simulink model "CNcs5"  (Simulink 6.2)
settings: Solver=ode4  SolverMode=SingleTasking  StartTime=0.0  StopTime=5  FixedStep=0.001  MaxStep=0.001  RelTol=1e-3  AbsTol=1e-3
undefined symbols (not defined in the file): alexlaw, bs_onoff, bs_scale, bsfsacrit, bsfsvcrit, cnsgain, fs_onoff, fs_scale, fsdelaycalc, ltdrk, phasicgain, pmcgain, pmctau2, pmctau3, saccrefract, saccsw, spgain, tonicgain, tvrD, tvrN, velnoise, velreconsw
libraries: simulink_extras x38, simulink x2
(part 1 of 5)
settings Model: Creator=jacobs  LastModifiedBy=jacobs  ExtModeAutoUpdateStatusClock=off
settings DataIOCC: LimitDataPoints=off  SaveOutput=off  SaveTime=off
settings OptimizationCC: BlockReduction=off  BooleanDataType=off
settings HardwareCC: TargetUnknown=on
settings STFCustomTargetCC: TargetFcnLib=ansi_tfl_tmw.mat  GenFloatMathFcnCalls=ANSI_C  ModelReferenceCompliant=off  SystemTargetFile=grt.tlc

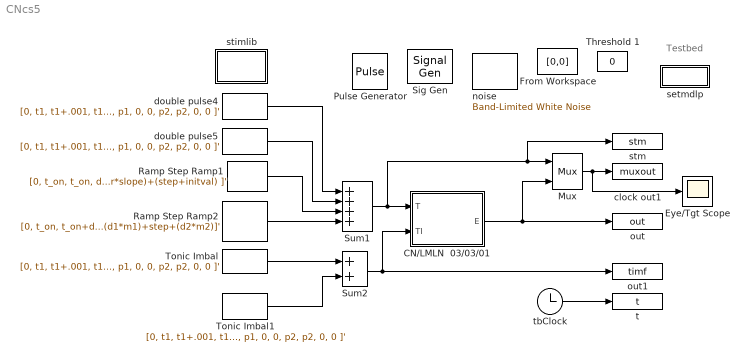
== system CNcs5 ==
  note: Testbed
  CN/LMLN  03/03/01 : Subsystem
      mask init:
      | k=0.25;loadmdlp;
      mask Display: disp('CN & LMLN\nModel')
  Eye/Tgt Scope : Scope
      settings: TickLabels=on  TimeRange=5  YMin=-5  YMax=32.5  DataFormat=Array
  From Workspace : FromWorkspace  VariableName=[0,0]
  Mux : Mux  Inputs=2
  Pulse Generator : DiscretePulseGenerator  PulseType=Time based  Amplitude=2  Period=.5  PulseWidth=100 * (.04)/(.5)  PhaseDelay=.1
  Ramp Step Ramp1 : FromWorkspace  VariableName=[0, t_on, t_on, dur+t_on dur+t_on; initval, initval, initval+step, (dur*slope)+(step+initval), (dur*slope)+(step+initval) ]'  mask{initval=0, t_on=1, step=0, dur=5, slope=0}
      mask prompts: initval "Initial value"; t_on "Time of step"; step "Size of step"; dur "Ramp duration"; slope "Ramp slope"
      mask help: Ramp Step Ramp
      mask Display: disp('Step\nRamp')
  Ramp Step Ramp2 : FromWorkspace  VariableName=[0, t_on, t_on+d1, t_on+d1, t_on+d1+d2, 10000; vi, vi, vi+(d1*m1), (vi+step)+(d1*m1), (vi+step)+(d1*m1)+(d2*m2), vi+(d1*m1)+step+(d2*m2)]'  mask{vi=0, t_on=.25, d1=4, m1=0, step=0, d2=2, m2=0}
      mask prompts: vi "Initial value"; t_on "Time of first ramp"; d1 "First Ramp duration"; m1 "First Ramp slope"; step "Size of step"; d2 "Second Ramp duration"; m2 "Second Ramp slope"
      mask help: Ramp Step Ramp
      mask Display: disp('Ramp\nStep\nRamp')
  Sig Gen : SignalGenerator  WaveForm=square  Amplitude=1.000000  Frequency=10.000000  Units=rad/sec
  Sum1 : Sum  Inputs=++++  SaturateOnIntegerOverflow=on  InputSameDT=on
  Sum2 : Sum  SaturateOnIntegerOverflow=on  InputSameDT=on
  Threshold 1 : Constant  Value=0
  Tonic Imbal : FromWorkspace  VariableName=[0, t1, t1+.001, t1+d1, t1+d1+.001, t1+d1+.001+ipd, t1+d1+.001+ipd, t1+d1+.001+ipd+d2, t1+d1+.001+ipd+d2, 10000; 0, 0, p1, p1, 0, 0, p2, p2, 0, 0 ]'  mask{@1=0, @2=0, @3=2, @4=0, @5=0, @6=3}
      mask prompts: @1 "Pulse 1 Magnitude"; @2 "Time of Pulse 1 Onset"; @3 "Pulse 1 Duration"; @4 "Interpulse Delay"; @5 "Pulse 2 Magnitude"; @6 "Pulse 2 Duration"
      mask help: Double Pulse
      mask init:
      | p1=@1; t1=@2; d1=@3; ipd=@4; p2=@5; d2=@6;
      mask Display: disp('Double\nPulse')
  Tonic Imbal1 : FromWorkspace  VariableName=[0, t1, t1+.001, t1+d1, t1+d1+.001, t1+d1+.001+ipd, t1+d1+.001+ipd, t1+d1+.001+ipd+d2, t1+d1+.001+ipd+d2, 10000; 0, 0, p1, p1, 0, 0, p2, p2, 0, 0 ]'  mask{@1=0, @2=0, @3=3.5, @4=0, @5=0, @6=1.5}
      mask prompts: @1 "Pulse 1 Magnitude"; @2 "Time of Pulse 1 Onset"; @3 "Pulse 1 Duration"; @4 "Interpulse Delay"; @5 "Pulse 2 Magnitude"; @6 "Pulse 2 Duration"
      mask help: Double Pulse
      mask init:
      | p1=@1; t1=@2; d1=@3; ipd=@4; p2=@5; d2=@6;
      mask Display: disp('Double\nPulse')
  clock out1 : ToWorkspace  VariableName=muxout  SaveFormat=Array
      settings: MaxDataPoints=100000
  double pulse4 : FromWorkspace  VariableName=[0, t1, t1+.001, t1+d1, t1+d1+.001, t1+d1+.001+ipd, t1+d1+.001+ipd, t1+d1+.001+ipd+d2, t1+d1+.001+ipd+d2, 10000; 0, 0, p1, p1, 0, 0, p2, p2, 0, 0 ]'  mask{@1=15, @2=2, @3=2, @4=0, @5=0, @6=5}
      mask prompts: @1 "Pulse 1 Magnitude"; @2 "Time of Pulse 1 Onset"; @3 "Pulse 1 Duration"; @4 "Interpulse Delay"; @5 "Pulse 2 Magnitude"; @6 "Pulse 2 Duration"
      mask help: Double Pulse
      mask init:
      | p1=@1; t1=@2; d1=@3; ipd=@4; p2=@5; d2=@6;
      mask Display: disp('Double\nPulse')
  double pulse5 : FromWorkspace  VariableName=[0, t1, t1+.001, t1+d1, t1+d1+.001, t1+d1+.001+ipd, t1+d1+.001+ipd, t1+d1+.001+ipd+d2, t1+d1+.001+ipd+d2, 10000; 0, 0, p1, p1, 0, 0, p2, p2, 0, 0 ]'  mask{@1=0, @2=0, @3=1, @4=0, @5=0, @6=4.5}
      mask prompts: @1 "Pulse 1 Magnitude"; @2 "Time of Pulse 1 Onset"; @3 "Pulse 1 Duration"; @4 "Interpulse Delay"; @5 "Pulse 2 Magnitude"; @6 "Pulse 2 Duration"
      mask help: Double Pulse
      mask init:
      | p1=@1; t1=@2; d1=@3; ipd=@4; p2=@5; d2=@6;
      mask Display: disp('Double\nPulse')
  noise : simulink/Sources/Band-Limited White Noise  Cov=[0.1]  Ts=0.1  seed=[23341]
  out : ToWorkspace  VariableName=out  SaveFormat=Array
      settings: MaxDataPoints=100000
  out1 : ToWorkspace  VariableName=timf  SaveFormat=Array
      settings: MaxDataPoints=100000
  setmdlp : Subsystem
      settings: OpenFcn=setmdlp
      mask Display: disp('setmdlp')
  stimlib : Subsystem
      settings: OpenFcn=stimlib
      mask Display: disp('Stimlib')
  stm : ToWorkspace  VariableName=stm  SaveFormat=Array
      settings: MaxDataPoints=100000
  t : ToWorkspace  VariableName=t  SaveFormat=Array
      mask init:
      | global t
      settings: MaxDataPoints=100000
  tbClock : Clock
      settings: Decimation=10
  wires:
  tbClock/1 -> t/1
  double pulse4/1 -> Sum1/1
  Sum1/1 -> CN/LMLN  03/03/01/1(T), stm/1, Mux/1
  CN/LMLN  03/03/01/1(E) -> out/1, Mux/2
  Mux/1 -> clock out1/1, Eye/Tgt Scope/1
  Tonic Imbal/1 -> Sum2/1
  Tonic Imbal1/1 -> Sum2/2
  Sum2/1 -> CN/LMLN  03/03/01/2(TI), out1/1
  double pulse5/1 -> Sum1/2
  Ramp Step Ramp1/1 -> Sum1/3
  Ramp Step Ramp2/1 -> Sum1/4

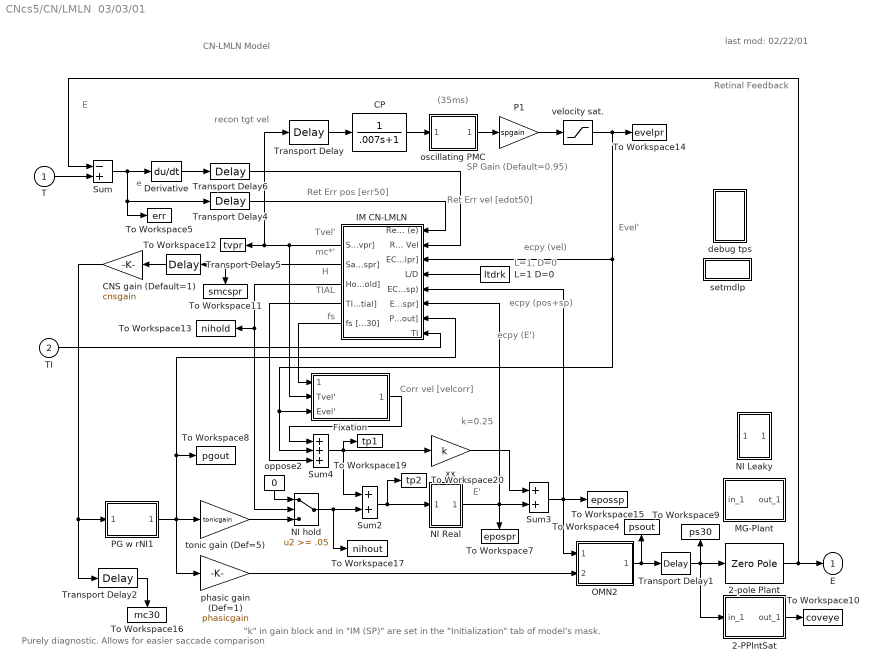
== system CNcs5/CN/LMLN  03/03/01 ==
  note: E'
  note: k=0.25
  note: "k" in gain block and in "IM (SP)" are set in
      | the "Initialization" tab of model's mask.
  note: E
  note: e
  note: TIAL
  note: H
  note: mc*'
  note: Tvel'
  note: ecpy
      | (E')
  note: ecpy (vel)
  note: (35ms)
  note: Retinal Feedback
  note: recon tgt vel
  note: last mod:
      | 02/22/01
  note: Evel'
  note: CN-LMLN Model
  note: ecpy
      | (pos+sp)
  note: Ret Err vel
      | [edot50]
  note: Ret Err pos [err50]
  note: Purely diagnostic.  Allows for easier
      | saccade comparison
  note: SP Gain
      | (Default=0.95)
  note: L=1, D=0
  note: Corr vel
      | [velcorr]
  note: fs
  T : Inport  Port=1  LatchInput=off
  TI : Inport  Port=2  LatchInput=off
  2-PPlntSat : Subsystem
      mask Display: disp('2-P Plant\n[Sat]')
  2-pole Plant : ZeroPole  Zeros=[ ]  Poles=[ -1/.18 -1/.007]  Gain=[1/.18 * 1/.007]
      mask Display: disp('2-pole\nPlant')
  CNS gain (Default=1) : Gain  Orientation=left  Gain=cnsgain  SaturateOnIntegerOverflow=on
  CP : TransferFcn  Denominator=[.007 1]
  Derivative : Derivative
      mask Display: disp('s')
  Fixation : Subsystem
      mask Display: disp('Fixation')
  IM CN-LMLN : Subsystem  Orientation=left
      mask Display: disp('IM\nCN-LMLN')
  L=1 D=0 : Constant  Orientation=left  Value=ltdrk
  MG-Plant : Subsystem
      mask Display: disp('MG Plant\n[K,tau,sat]')
  NI Leaky : Subsystem
      mask Display: disp('N\nLeaky')
  NI Real : Subsystem
      mask Display: disp('NI\nReal')
  NI hold : Switch  Threshold=.05  SaturateOnIntegerOverflow=on  InputSameDT=on
  OMN2 : Subsystem
      mask Display: disp('<--"tonic" \nOMN2\n<--"phasic"')
  P1 : Gain  Gain=spgain  SaturateOnIntegerOverflow=on
  PG w rNI1 : Subsystem
      mask Display: disp('PG rNI\n(2P)')
  Sum : Sum  Inputs=-+  SaturateOnIntegerOverflow=on  InputSameDT=on
  Sum2 : Sum  SaturateOnIntegerOverflow=on  InputSameDT=on
  Sum3 : Sum  SaturateOnIntegerOverflow=on  InputSameDT=on
  Sum4 : Sum  Inputs=+++  SaturateOnIntegerOverflow=on  InputSameDT=on
  To Workspace10 : ToWorkspace  VariableName=coveye  SaveFormat=Array
      settings: MaxDataPoints=10000
  To Workspace11 : ToWorkspace  VariableName=smcspr  SaveFormat=Array
      settings: Orientation=down  MaxDataPoints=10000
  To Workspace12 : ToWorkspace  VariableName=tvpr  SaveFormat=Array
      settings: MaxDataPoints=10000
  To Workspace13 : ToWorkspace  VariableName=nihold  SaveFormat=Array
      settings: MaxDataPoints=10000
  To Workspace14 : ToWorkspace  VariableName=evelpr  SaveFormat=Array
      settings: MaxDataPoints=10000
  To Workspace15 : ToWorkspace  VariableName=epossp  SaveFormat=Array
      settings: MaxDataPoints=10000
  To Workspace16 : ToWorkspace  VariableName=mc30  SaveFormat=Array
      settings: Orientation=down  MaxDataPoints=10000
  To Workspace17 : ToWorkspace  VariableName=nihout  SaveFormat=Array
      settings: MaxDataPoints=10000
  To Workspace19 : ToWorkspace  VariableName=tp1  SaveFormat=Array
      settings: MaxDataPoints=10000
  To Workspace20 : ToWorkspace  VariableName=tp2  SaveFormat=Array
      settings: MaxDataPoints=10000
  To Workspace4 : ToWorkspace  VariableName=psout  SaveFormat=Array
      settings: Orientation=up  MaxDataPoints=10000
  To Workspace5 : ToWorkspace  VariableName=err  SaveFormat=Array
      settings: MaxDataPoints=10000
  To Workspace7 : ToWorkspace  VariableName=epospr  SaveFormat=Array
      settings: Orientation=down  MaxDataPoints=10000
  To Workspace8 : ToWorkspace  VariableName=pgout  SaveFormat=Array
      settings: MaxDataPoints=10000
  To Workspace9 : ToWorkspace  VariableName=ps30  SaveFormat=Array
      settings: Orientation=up  MaxDataPoints=10000
  Transport Delay : TransportDelay  DelayTime=0.015
      mask Display: disp('15ms')
  Transport Delay1 : TransportDelay  DelayTime=0.03
      mask Display: disp('30ms')
  Transport Delay2 : TransportDelay  DelayTime=0.03
      mask Display: disp('30ms')
  Transport Delay4 : TransportDelay  DelayTime=.05
      mask Display: disp('50ms')
  Transport Delay5 : TransportDelay  Orientation=left  DelayTime=0.001
      mask Display: disp('1ms')
  Transport Delay6 : TransportDelay  DelayTime=.05
      mask Display: disp('50ms')
  debug tps : Subsystem
  oppose2 : Constant  Orientation=down  Value=0
  oscillating PMC : Subsystem
      mask Display: disp('PMC+')
  phasic gain (Def=1) : Gain  Gain=phasicgain  SaturateOnIntegerOverflow=on
  setmdlp : Subsystem
      settings: OpenFcn=setmdlp
      mask Display: disp('setmdlp')
  tonic gain (Def=5) : Gain  Gain=tonicgain  SaturateOnIntegerOverflow=on
  velocity sat. : Saturate  UpperLimit=90  LowerLimit=-90
  xx : Gain  Gain=k  SaturateOnIntegerOverflow=on
  E : Outport  InitialOutput=0
  wires:
  Derivative/1 -> Transport Delay6/1
  Sum/1 -> Derivative/1, Transport Delay4/1, To Workspace5/1
  T/1 -> Sum/2
  Transport Delay4/1 -> IM CN-LMLN/1(RetErr Pos (e))
  L=1 D=0/1 -> IM CN-LMLN/4(L/D)
  Transport Delay6/1 -> IM CN-LMLN/2(RetErr Vel)
  CP/1 -> oscillating PMC/1(desired eye vel)
  oscillating PMC/1(efference copy eye vel) -> P1/1
  Transport Delay/1 -> CP/1
  velocity sat./1 -> To Workspace14/1, IM CN-LMLN/3(ECPY [evelpr]), Fixation/3(Evel'), Sum4/2
  P1/1 -> velocity sat./1
  TI/1 -> IM CN-LMLN/8(TI)
  IM CN-LMLN/1(SPmc [tvpr]) -> To Workspace12/1, Transport Delay/1, Fixation/2(Tvel')
  Sum4/1 -> xx/1, Sum2/1, To Workspace19/1
  IM CN-LMLN/4(TIAL [tial]) -> Sum4/3
  PG w rNI1/1(PG [pgout]) -> IM CN-LMLN/7(PG [pgout]), To Workspace8/1, tonic gain (Def=5)/1, phasic gain (Def=1)/1
  2-pole Plant/1 -> E/1, Sum/1
  2-PPlntSat/1(out_1) -> To Workspace10/1
  Transport Delay1/1 -> 2-pole Plant/1, To Workspace9/1, 2-PPlntSat/1(in_1)
  OMN2/1("[psout]") -> To Workspace4/1, Transport Delay1/1
  Transport Delay2/1 -> To Workspace16/1
  tonic gain (Def=5)/1 -> NI hold/3
  phasic gain (Def=1)/1 -> OMN2/2("[pgout]")
  NI hold/1 -> Sum2/2, To Workspace17/1
  xx/1 -> Sum3/1
  NI Real/1(NIOUT [epospr]) -> Sum3/2, To Workspace7/1, IM CN-LMLN/6(ECPY [epospr])
  Sum3/1 -> IM CN-LMLN/5(ECPY (epossp)), To Workspace15/1, OMN2/1("[epossp]")
  Fixation/1(" CorrVel [velcorr]") -> Sum4/1
  Sum2/1 -> NI Real/1(PG + (TIAL+SP)), To Workspace20/1
  IM CN-LMLN/5(fs [fsmc30]) -> Fixation/1(fs [fsmc30])
  oppose2/1 -> NI hold/1
  IM CN-LMLN/3(Hold [nihold]) -> To Workspace13/1, NI hold/2
  IM CN-LMLN/2(Saccmc [smcspr]) -> To Workspace11/1, Transport Delay5/1
  CNS gain (Default=1)/1 -> PG w rNI1/1("[mcsprd]"), Transport Delay2/1
  Transport Delay5/1 -> CNS gain (Default=1)/1

== system CNcs5/setmdlp ==

== system CNcs5/stimlib ==

== system CNcs5/CN/LMLN  03/03/01/2-PPlntSat ==
  note: A 2-pole plant can be simulated by:
      | 1. no limitation on lateral gaze
      | 2. a hard limitation - placing a saturation in the plant [eg, 55 deg]
      | 3. a soft limitation - add the dead zone  [DZ slope>0]
  in_1 : Inport  Port=1  LatchInput=off
  2 pole : ZeroPole  Zeros=[ ]  Poles=[ -1/.18 -1/.007]  Gain=[1/.18 * 1/.007]
      mask Display: disp('2-pole\nPlant')
  DZ slope : Constant  Value=0.05
  Dead Zone : DeadZone  LowerValue=-55  UpperValue=55  SaturateOnIntegerOverflow=on
  Product : Product  SaturateOnIntegerOverflow=on  RndMeth=Zero  InputSameDT=on
  Saturation : Saturate  UpperLimit=55  LowerLimit=-55
  Sum3 : Sum  SaturateOnIntegerOverflow=on  InputSameDT=on
  out_1 : Outport  InitialOutput=0
  wires:
  DZ slope/1 -> Product/2
  Product/1 -> Sum3/2
  Sum3/1 -> out_1/1
  Saturation/1 -> Sum3/1
  Dead Zone/1 -> Product/1
  2 pole/1 -> Saturation/1, Dead Zone/1
  in_1/1 -> 2 pole/1

== system CNcs5/CN/LMLN  03/03/01/Fixation ==
  note: Fixation (counter-signal)
  note: Last mod: 02/22/01
  note: Positional error is passed through a gaussian-like function whose greatest
      | response occurs between +/-0.5 deg (approx), corresponding to the sensitivity
      | of the fovea.
  note: This factor is used (with an additional gain factor) to scale the velocity error,
      | which is then subtracted from the velocity signal that is sent from the
      | common neural integrator to the ocular motor neurons.
  note: This should have the effect of reducing the high velocity error (due
      | to CN oscillation or other sources) enough to permit an extension of
      | the foveation period.
  note: *Mod*
  fs [fsmc30] : Inport  Port=1  LatchInput=off
  Tvel' : Inport  Port=2  LatchInput=off
  Evel' : Inport  Port=3  LatchInput=off
  "30 " : Subsystem  mask{prolong=30}
      mask prompts: prolong "Prolong pulse by?  (msec)"
      mask Display: disp('prolong')
  Boolify2 : Subsystem
      mask Display: disp('Boolify')
  Product : Product  Inputs=3  SaturateOnIntegerOverflow=on  RndMeth=Zero  InputSameDT=on
  Product1 : Product  SaturateOnIntegerOverflow=on  RndMeth=Zero  InputSameDT=on
  Sum5 : Sum  Inputs=+-  SaturateOnIntegerOverflow=on  InputSameDT=on
  Transport Delay7 : TransportDelay  DelayTime=0.050
      mask Display: disp('50ms')
  Vel Sens Factor : Gain  Gain=4  SaturateOnIntegerOverflow=on
  WF % to be applied : Gain  SaturateOnIntegerOverflow=on
  on/off : Constant  Orientation=down
  position sensitivity W2 : Lookup  InputValues="[-5 -2  -1 -0.5   0.5   1    2    5]"  OutputValues="[ 0   0.125    0.5     1      1     0.5    0.125  0]"  SaturateOnIntegerOverflow=on
  t : ToWorkspace  VariableName=velfact  SaveFormat=Array
      mask init:
      | global t
      settings: MaxDataPoints=100000
  t2 : ToWorkspace  VariableName=velcorr  SaveFormat=Array
      mask init:
      | global t
      settings: MaxDataPoints=100000
  t3 : ToWorkspace  VariableName=fs30p  SaveFormat=Array
      mask init:
      | global t
      settings: MaxDataPoints=100000
  t4 : ToWorkspace  VariableName=nystagvel  SaveFormat=Array
      mask init:
      | global t
      settings: MaxDataPoints=100000
  velocity sensitivity N : Lookup  InputValues="[-20 -16  -12   -6  -4  4   6   12  16 20]"  OutputValues="[0 0   0.1    0.3    1   1   0.3  0.1   0 0]"  SaturateOnIntegerOverflow=on
  velocity sensitivity W2 : Lookup  InputValues="[-30 -15   -8  -4   4     8  15  30]"  OutputValues="[0  0.125   0.5    1    1    0.5   0.125  0]"  SaturateOnIntegerOverflow=on
  " CorrVel [velcorr]" : Outport  InitialOutput=0
  wires:
  Sum5/1 -> velocity sensitivity N/1, t4/1, WF % to be applied/1
  velocity sensitivity N/1 -> Vel Sens Factor/1, t/1
  Evel'/1 -> Sum5/2
  Tvel'/1 -> Transport Delay7/1
  Transport Delay7/1 -> Sum5/1
  WF % to be applied/1 -> Product/3
  Product/1 -> t2/1, Product1/2
  Product1/1 -> " CorrVel [velcorr]"/1
  on/off/1 -> Product1/1
  fs [fsmc30]/1 -> Boolify2/1(In1)
  Boolify2/1(Out1) -> "30 "/1(value(in))
  "30 "/1(value(out)) -> Product/1, t3/1
  Vel Sens Factor/1 -> Product/2

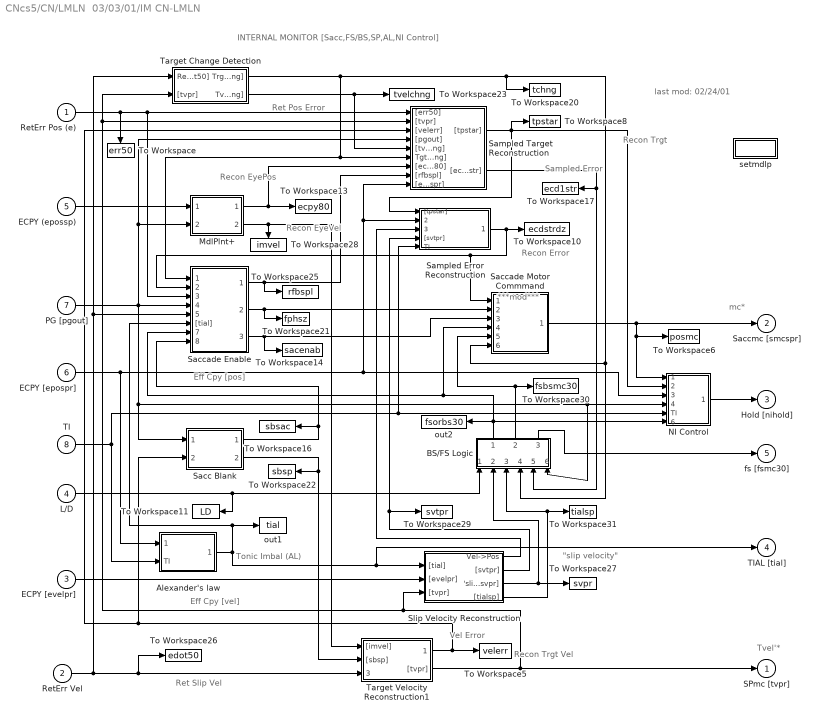
== system CNcs5/CN/LMLN  03/03/01/IM CN-LMLN ==
  note: INTERNAL MONITOR [Sacc,FS/BS,SP,AL,NI Control]
  note: last mod:
      | 02/24/01
  note: mc*
  note: Tvel'*
  note: "slip velocity"
  note: Recon
      | Trgt
  note: Recon
      | EyePos
  note: Recon
      | EyeVel
  note: Sampled
      | Error
  note: Recon Error
  note: Recon
      | Trgt Vel
  note: Vel
      | Error
  note: Eff Cpy [vel]
  note: Eff Cpy [pos]
  note: Tonic Imbal (AL)
  note: Ret Slip Vel
  note: Ret Pos Error
  note: ***mod***
  RetErr Pos (e) : Inport  Port=1  LatchInput=off
  RetErr Vel : Inport  Port=2  LatchInput=off
  ECPY [evelpr] : Inport  Port=3  LatchInput=off
  L/D : Inport  Port=4  LatchInput=off
  ECPY (epossp) : Inport  Port=5  LatchInput=off
  ECPY [epospr] : Inport  Port=6  LatchInput=off
  PG [pgout] : Inport  Port=7  LatchInput=off
  TI : Inport  Port=8  LatchInput=off
  Alexander's law : Subsystem  mask{slope=alexlaw}
      mask help: Alexander's Law
      mask Display: disp('Alexander''s\nLaw')
  BS/FS Logic : Subsystem  Orientation=up
      mask Display: disp('BS/FS\nLogic')
  MdlPlnt+ : Subsystem
      mask Display: disp('Model\nPlant+')
  NI Control : Subsystem
      mask Display: disp('NI\nControl')
  Sacc Blank : Subsystem
      mask Display: disp('Saccade\n& Drift\nBlanking')
  Saccade Enable : Subsystem
      mask Display: disp('Saccade\nEnable')
  Saccade Motor Commmand : Subsystem
      mask Display: disp('Saccade\nMotor\nCommand')
  Sampled Error Reconstruction : Subsystem
      mask Display: disp('Sampled Error\nReconstruction')
  Sampled Target Reconstruction : Subsystem
      mask Display: disp('Sampled\nTarget\nReconstruction')
  Slip Velocity Reconstruction : Subsystem
      mask Display: disp('Slip\nVelocity\nReconstruction')
  Target Change Detection : Subsystem
      mask Display: disp('Target Change\nDetection')
  Target Velocity Reconstruction1 : Subsystem
      mask Display: disp('Target\nVelocity\nReconstruction')
  To Workspace : ToWorkspace  VariableName=err50  SaveFormat=Array
      settings: Orientation=down  MaxDataPoints=10000
  To Workspace10 : ToWorkspace  VariableName=ecdstrdz  SaveFormat=Array
      settings: MaxDataPoints=10000
  To Workspace11 : ToWorkspace  VariableName=LD  SaveFormat=Array
      settings: MaxDataPoints=10000
  To Workspace13 : ToWorkspace  VariableName=ecpy80  SaveFormat=Array
      settings: MaxDataPoints=10000
  To Workspace14 : ToWorkspace  VariableName=sacenab  SaveFormat=Array
      settings: MaxDataPoints=10000
      mask Type: imsw1in
  To Workspace16 : ToWorkspace  VariableName=sbsac  SaveFormat=Array
      settings: MaxDataPoints=10000
  To Workspace17 : ToWorkspace  VariableName=ecd1str  SaveFormat=Array
      settings: MaxDataPoints=10000
  To Workspace20 : ToWorkspace  VariableName=tchng  SaveFormat=Array
      settings: MaxDataPoints=10000
  To Workspace21 : ToWorkspace  VariableName=fphsz  SaveFormat=Array
      settings: MaxDataPoints=10000
  To Workspace22 : ToWorkspace  VariableName=sbsp  SaveFormat=Array
      settings: MaxDataPoints=10000
  To Workspace23 : ToWorkspace  VariableName=tvelchng  SaveFormat=Array
      settings: MaxDataPoints=10000
  To Workspace25 : ToWorkspace  VariableName=rfbspl  SaveFormat=Array
      settings: MaxDataPoints=10000
      mask Type: imsw1in
  To Workspace26 : ToWorkspace  VariableName=edot50  SaveFormat=Array
      settings: MaxDataPoints=10000
  To Workspace27 : ToWorkspace  VariableName=svpr  SaveFormat=Array
      settings: MaxDataPoints=10000
  To Workspace28 : ToWorkspace  VariableName=imvel  SaveFormat=Array
      settings: Orientation=down  MaxDataPoints=10000
      mask Type: imsw1in
  To Workspace29 : ToWorkspace  VariableName=svtpr  SaveFormat=Array
      settings: MaxDataPoints=10000
  To Workspace30 : ToWorkspace  VariableName=fsbsmc30  SaveFormat=Array
      settings: MaxDataPoints=10000
  To Workspace31 : ToWorkspace  VariableName=tialsp  SaveFormat=Array
      settings: MaxDataPoints=10000
  To Workspace5 : ToWorkspace  VariableName=velerr  SaveFormat=Array
      settings: MaxDataPoints=10000
  To Workspace6 : ToWorkspace  VariableName=posmc  SaveFormat=Array
      settings: MaxDataPoints=10000
  To Workspace8 : ToWorkspace  VariableName=tpstar  SaveFormat=Array
      settings: MaxDataPoints=10000
  out1 : ToWorkspace  VariableName=tial  SaveFormat=Array
      settings: MaxDataPoints=100000
  out2 : ToWorkspace  VariableName=fsorbs30  SaveFormat=Array
      settings: MaxDataPoints=100000
  setmdlp : Subsystem
      settings: OpenFcn=setmdlp
      mask Display: disp('setmdlp')
  SPmc [tvpr] : Outport  InitialOutput=0
  Saccmc [smcspr] : Outport  Port=2  InitialOutput=0
  Hold [nihold] : Outport  Port=3  InitialOutput=0
  TIAL [tial] : Outport  Port=4  InitialOutput=0
  fs [fsmc30] : Outport  Port=5  InitialOutput=0
  wires:
  NI Control/1(Hold [nihold]) -> Hold [nihold]/1
  L/D/1 -> BS/FS Logic/1(L/D), To Workspace11/1
  ECPY [epospr]/1 -> Alexander's law/1(ECPY [epospr]), NI Control/3("[epospr]"), Sampled Error Reconstruction/2("[epospr]"), Sampled Target Reconstruction/9("[epospr]")
  TI/1 -> Alexander's law/2(TI), NI Control/5(TI), Sampled Error Reconstruction/5(TI)
  PG [pgout]/1 -> Sacc Blank/1(PG [pgout]), NI Control/4(PG [pgout]), BS/FS Logic/6("[pgout]"), Saccade Enable/4("[pgout]"), MdlPlnt+/2("[pgout]"), Sampled Target Reconstruction/4("[pgout]")
  ECPY (epossp)/1 -> MdlPlnt+/1("[epossp]")
  MdlPlnt+/2("[imvel]") -> To Workspace28/1, Target Velocity Reconstruction1/1("[imvel]")
  BS/FS Logic/1("[fsorbs30]") -> out2/1, Saccade Enable/7("[fsorbs30]"), Saccade Motor Commmand/4("[fsorbs30]"), NI Control/6("[fsorbs30]")
  Saccade Enable/2(FPh Size [fphsz]) -> To Workspace21/1, Saccade Motor Commmand/2("[fphsz]")
  Saccade Enable/3("[sacenab]") -> To Workspace14/1, Saccade Motor Commmand/3("[sacenab]")
  Saccade Enable/1("[rfbspl]") -> To Workspace25/1, Sampled Target Reconstruction/8("[rfbspl]")
  MdlPlnt+/1("[ecpy80]") -> Sampled Target Reconstruction/7("[ecpy80]"), To Workspace13/1
  Sacc Blank/2(SP S/H [sbsp]) -> Target Velocity Reconstruction1/2("[sbsp]"), To Workspace22/1
  Alexander's law/1(TIAL [tial]) -> Saccade Enable/6("[tial]"), out1/1, Slip Velocity Reconstruction/1("[tial]"), TIAL [tial]/1
  Saccade Motor Commmand/1("[posmc]") -> NI Control/1("[posmc]"), To Workspace6/1, Saccmc [smcspr]/1
  Slip Velocity Reconstruction/1(Vel->Pos) -> Sampled Error Reconstruction/3((sv+tial) k)
  Slip Velocity Reconstruction/2("[svtpr]") -> Sampled Error Reconstruction/4("[svtpr]"), To Workspace29/1
  Slip Velocity Reconstruction/3("'slip vel\" [svpr]") -> BS/FS Logic/2(slip vel [svpr]), To Workspace27/1
  Target Change Detection/1(Trgt Chng [tchng]) -> Sampled Target Reconstruction/6(Tgt ch Det [tchng]), Saccade Enable/1(Tgt ch Det [tchng]), BS/FS Logic/4(Tgt ch Det [tchng]), Saccade Motor Commmand/6(Tgt ch Det [tchng]), To Workspace20/1
  Sampled Target Reconstruction/1("[tpstar]") -> To Workspace8/1, Sampled Error Reconstruction/1("[tpstar]"), NI Control/2(T'* [tpstar])
  ECPY [evelpr]/1 -> Slip Velocity Reconstruction/2("[evelpr]")
  RetErr Pos (e)/1 -> To Workspace/1, Saccade Enable/3("[err50]"), Sampled Target Reconstruction/1("[err50]")
  Target Change Detection/2(Tvel Chng [tvelchng]) -> To Workspace23/1, Sampled Target Reconstruction/5("[tvelchng]")
  RetErr Vel/1 -> Target Velocity Reconstruction1/3("[edot50]"), To Workspace26/1, Target Change Detection/1(RetErr Vel [edot50]), Saccade Enable/5("[edot50]")
  Target Velocity Reconstruction1/1("[velerr]") -> To Workspace5/1, Sacc Blank/2(RetVelErr [velerr]), Sampled Target Reconstruction/3("[velerr]")
  Target Velocity Reconstruction1/2("[tvpr]") -> SPmc [tvpr]/1, Slip Velocity Reconstruction/3("[tvpr]"), Target Change Detection/2("[tvpr]"), Sampled Target Reconstruction/2("[tvpr]")
  Sacc Blank/1(SacBlnk [sbsac]) -> Saccade Enable/8("[sbsac]"), To Workspace16/1
  Slip Velocity Reconstruction/4("[tialsp]") -> BS/FS Logic/3(Evel' [evelpr]), To Workspace31/1
  Sampled Error Reconstruction/1("[ecdstrdz] (excl nystag)") -> To Workspace10/1, Saccade Motor Commmand/1("[ecdstrdz]"), Saccade Enable/2("[ecdstrdz]")
  Sampled Target Reconstruction/2("[ecd1str]") -> BS/FS Logic/5(ECD1* [ecd1str]), To Workspace17/1
  BS/FS Logic/2("[fsbsmc30]") -> Saccade Motor Commmand/5("[fsbcmc30]"), To Workspace30/1
  BS/FS Logic/3("[fsmc30]") -> fs [fsmc30]/1

== system CNcs5/CN/LMLN  03/03/01/MG-Plant ==
  note: Place MG Plant as fixating eye and feed output of normal plant to a testpoint [eg, coveye]
  note: MG can be simulated by:
      | 1. a staticgain deficit -  reducing the plant gain (P) [eg, gain P=0.6]
      | 2. a tonic gain deficit - reducing the effective time constant of the plant [eg, gain K=0.6]
      | 3. a hard paresis - placing a saturation in the plant [eg, 5 - 20 deg]
      | 4. a soft paresis - add the dead zone  [DZ slope>0]
  in_1 : Inport  Port=1  LatchInput=off
  2 pole : ZeroPole  Zeros=[ ]  Poles=[ -1/.18 -1/.007]  Gain=[1/.18 * 1/.007]
      mask Display: disp('2-pole\nPlant')
  DZ slope : Constant  Value=0
  Dead Zone : DeadZone  LowerValue=-5  UpperValue=12  SaturateOnIntegerOverflow=on
  Gain P : Gain  Gain=0.3  SaturateOnIntegerOverflow=on
  GainK : Gain  Orientation=left  Gain=0  SaturateOnIntegerOverflow=on
  Product : Product  SaturateOnIntegerOverflow=on  RndMeth=Zero  InputSameDT=on
  Saturation : Saturate  UpperLimit=50  LowerLimit=-50
  Sum2 : Sum  Inputs=+-  SaturateOnIntegerOverflow=on  InputSameDT=on
  Sum3 : Sum  SaturateOnIntegerOverflow=on  InputSameDT=on
  out_1 : Outport  InitialOutput=0
  wires:
  GainK/1 -> Sum2/2
  in_1/1 -> Sum2/1
  Sum2/1 -> Gain P/1
  Gain P/1 -> 2 pole/1
  2 pole/1 -> Saturation/1, GainK/1, Dead Zone/1
  Dead Zone/1 -> Product/1
  Saturation/1 -> Sum3/1
  Sum3/1 -> out_1/1
  Product/1 -> Sum3/2
  DZ slope/1 -> Product/2

== system CNcs5/CN/LMLN  03/03/01/NI Leaky ==
  note: Neural Integrator Leaky
  in_1 : Inport  Port=1  LatchInput=off
  Constant : Constant
  Constant1 : Constant  Value=0
  Gain : Gain  Gain=0.05  SaturateOnIntegerOverflow=on
  Leak -50 : TransferFcn  Numerator=20  Denominator=[1 20]
  NI Real : Subsystem
      mask Display: disp('NI Real')
  Product : Product  SaturateOnIntegerOverflow=on  RndMeth=Zero  InputSameDT=on
  Product1 : Product  SaturateOnIntegerOverflow=on  RndMeth=Zero  InputSameDT=on
  Sum : Sum  SaturateOnIntegerOverflow=on  InputSameDT=on
  out_1 : Outport  InitialOutput=0
  wires:
  Sum/1 -> out_1/1
  Product1/1 -> Sum/2
  Gain/1 -> Leak -50/1
  in_1/1 -> Gain/1, NI Real/1(in_1)
  Leak -50/1 -> Product1/2
  Constant1/1 -> Product1/1
  Product/1 -> Sum/1
  NI Real/1(out_1) -> Product/1
  Constant/1 -> Product/2

== system CNcs5/CN/LMLN  03/03/01/NI Real ==
  note: NI Real
  PG + (TIAL+SP) : Inport  Port=1  LatchInput=off
  Gain : Gain  Gain=25  SaturateOnIntegerOverflow=on
  Gain1 : Gain  Orientation=left  SaturateOnIntegerOverflow=on
  Sum : Sum  SaturateOnIntegerOverflow=on  InputSameDT=on
  Transfer Fcn : TransferFcn  Numerator=[1/25]  Denominator=[1 1/25]
  NIOUT [epospr] : Outport  InitialOutput=0
  wires:
  PG + (TIAL+SP)/1 -> Gain/1
  Gain/1 -> Sum/2
  Sum/1 -> Transfer Fcn/1
  Gain1/1 -> Sum/1
  Transfer Fcn/1 -> Gain1/1, NIOUT [epospr]/1

== system CNcs5/CN/LMLN  03/03/01/OMN2 ==
  note: OMN
  note: Note that the OMN properly combines the pulse with the output of the NI, by latching
      | that output to its value at the moment the pulse appears.
  note: Operation: when the pulse is active ("from PG") it activates the switch, passing the
      | upper input through to the output.  When the pulse is over, the switch changes,
      | allowing the lower input (from the NI) to pass.
  note: This block behaves like the ocular motor neurons,combining a phasic pulse (from PG)
      | with the tonic step produced by integration of the step, yielding a Pulse-Step
      | to drive the plant.
  "[epossp]" : Inport  Port=1  LatchInput=off
  "[pgout]" : Inport  Port=2  LatchInput=off
  Abs : Abs  SaturateOnIntegerOverflow=on
  Gain _ : Gain  Gain=1.0  SaturateOnIntegerOverflow=on
  SampHold? : Subsystem
      mask Display: disp('H=H\nS=L')
  Sign : Signum
  Sum : Sum  SaturateOnIntegerOverflow=on  InputSameDT=on
  Switch : Switch  Threshold=.5  SaturateOnIntegerOverflow=on  InputSameDT=on
  "[psout]" : Outport  InitialOutput=0
  wires:
  "[epossp]"/1 -> Switch/3, SampHold?/1(Input)
  Sign/1 -> Switch/2, SampHold?/2(S/H?)
  Gain _/1 -> Sum/1
  SampHold?/1(output) -> Sum/2
  Sum/1 -> Switch/1
  "[pgout]"/1 -> Abs/1, Gain _/1
  Switch/1 -> "[psout]"/1
  Abs/1 -> Sign/1

== system CNcs5/CN/LMLN  03/03/01/PG w rNI1 ==
  note: Here it is at last!  A pulse generator based on a resettable integrator (look inside the PW
      | block).  The PW function controls the switch, allowing the output of the PH function to pass
      | for the appropriate duration.
  note: The refractory latch prevents the pulse generator from responding to another stimulus until a
      | physiologically acceptable refractory period has elapsed by controlling the "Sample and Hold" block.
  note: PG with Resettable NI
  note: (Init input:0)
  "[mcsprd]" : Inport  Port=1  LatchInput=off
  Constant1 : Constant  Orientation=up  Value=0
  PH funct : MATLABFcn  MATLABFcn=PHfn_ss
      mask Display: disp('PH\nfunction')
  PW funct : Subsystem
      mask Display: disp('PW\nfunction')
  RefLatch (Default = 50ms) : Subsystem  Orientation=left  mask{@1=saccrefract}
      mask prompts: @1 "Refractory Period (ms)"
      mask help: Refractory Latch
      mask init:
      | delay=@1;
      mask Display: disp('Refract\nLatch')
  SampHold?1 : Subsystem
      mask Display: disp('S=H\nH=L')
  Switch : Switch  Threshold=0.5  SaturateOnIntegerOverflow=on  InputSameDT=on
  To Workspace : ToWorkspace  VariableName=pgpk  SaveFormat=Array
      settings: Orientation=down  MaxDataPoints=10000
  To Workspace1 : ToWorkspace  VariableName=pgw  SaveFormat=Array
      settings: MaxDataPoints=10000
  To Workspace4 : ToWorkspace  VariableName=mcspl  SaveFormat=Array
      settings: MaxDataPoints=10000
  To Workspace5 : ToWorkspace  VariableName=refl  SaveFormat=Array
      settings: Orientation=down  MaxDataPoints=10000
  loop breaker : Memory  Orientation=left
  PG [pgout] : Outport  InitialOutput=0
  wires:
  PH funct/1 -> Switch/1, To Workspace/1
  PW funct/1(pgw) -> Switch/2, To Workspace1/1
  Constant1/1 -> Switch/3
  Switch/1 -> loop breaker/1, PG [pgout]/1
  loop breaker/1 -> RefLatch (Default = 50ms)/1(in_1)
  RefLatch (Default = 50ms)/1(out_1) -> SampHold?1/2(S/H?), To Workspace5/1
  SampHold?1/1(output) -> PH funct/1, PW funct/1(mcspl), To Workspace4/1
  "[mcsprd]"/1 -> SampHold?1/1(Input)

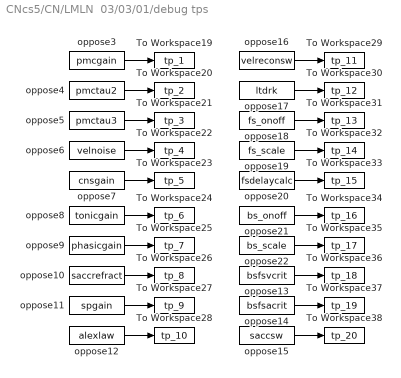
== system CNcs5/CN/LMLN  03/03/01/debug tps ==
  To Workspace19 : ToWorkspace  VariableName=tp_1  SaveFormat=Array
      settings: MaxDataPoints=10000
  To Workspace20 : ToWorkspace  VariableName=tp_2  SaveFormat=Array
      settings: MaxDataPoints=10000
  To Workspace21 : ToWorkspace  VariableName=tp_3  SaveFormat=Array
      settings: MaxDataPoints=10000
  To Workspace22 : ToWorkspace  VariableName=tp_4  SaveFormat=Array
      settings: MaxDataPoints=10000
  To Workspace23 : ToWorkspace  VariableName=tp_5  SaveFormat=Array
      settings: MaxDataPoints=10000
  To Workspace24 : ToWorkspace  VariableName=tp_6  SaveFormat=Array
      settings: MaxDataPoints=10000
  To Workspace25 : ToWorkspace  VariableName=tp_7  SaveFormat=Array
      settings: MaxDataPoints=10000
  To Workspace26 : ToWorkspace  VariableName=tp_8  SaveFormat=Array
      settings: MaxDataPoints=10000
  To Workspace27 : ToWorkspace  VariableName=tp_9  SaveFormat=Array
      settings: MaxDataPoints=10000
  To Workspace28 : ToWorkspace  VariableName=tp_10  SaveFormat=Array
      settings: MaxDataPoints=10000
  To Workspace29 : ToWorkspace  VariableName=tp_11  SaveFormat=Array
      settings: MaxDataPoints=10000
  To Workspace30 : ToWorkspace  VariableName=tp_12  SaveFormat=Array
      settings: MaxDataPoints=10000
  To Workspace31 : ToWorkspace  VariableName=tp_13  SaveFormat=Array
      settings: MaxDataPoints=10000
  To Workspace32 : ToWorkspace  VariableName=tp_14  SaveFormat=Array
      settings: MaxDataPoints=10000
  To Workspace33 : ToWorkspace  VariableName=tp_15  SaveFormat=Array
      settings: MaxDataPoints=10000
  To Workspace34 : ToWorkspace  VariableName=tp_16  SaveFormat=Array
      settings: MaxDataPoints=10000
  To Workspace35 : ToWorkspace  VariableName=tp_17  SaveFormat=Array
      settings: MaxDataPoints=10000
  To Workspace36 : ToWorkspace  VariableName=tp_18  SaveFormat=Array
      settings: MaxDataPoints=10000
  To Workspace37 : ToWorkspace  VariableName=tp_19  SaveFormat=Array
      settings: MaxDataPoints=10000
  To Workspace38 : ToWorkspace  VariableName=tp_20  SaveFormat=Array
      settings: MaxDataPoints=10000
  oppose10 : Constant  Value=saccrefract
  oppose11 : Constant  Value=spgain
  oppose12 : Constant  Value=alexlaw
  oppose13 : Constant  Value=bsfsvcrit
  oppose14 : Constant  Value=bsfsacrit
  oppose15 : Constant  Value=saccsw
  oppose16 : Constant  Value=velreconsw
  oppose17 : Constant  Value=ltdrk
  oppose18 : Constant  Value=fs_onoff
  oppose19 : Constant  Value=fs_scale
  oppose20 : Constant  Value=fsdelaycalc
  oppose21 : Constant  Value=bs_onoff
  oppose22 : Constant  Value=bs_scale
  oppose3 : Constant  Value=pmcgain
  oppose4 : Constant  Value=pmctau2
  oppose5 : Constant  Value=pmctau3
  oppose6 : Constant  Value=velnoise
  oppose7 : Constant  Value=cnsgain
  oppose8 : Constant  Value=tonicgain
  oppose9 : Constant  Value=phasicgain
  wires:
  oppose5/1 -> To Workspace21/1
  oppose8/1 -> To Workspace24/1
  oppose7/1 -> To Workspace23/1
  oppose6/1 -> To Workspace22/1
  oppose4/1 -> To Workspace20/1
  oppose3/1 -> To Workspace19/1
  oppose11/1 -> To Workspace27/1
  oppose12/1 -> To Workspace28/1
  oppose10/1 -> To Workspace26/1
  oppose9/1 -> To Workspace25/1
  oppose18/1 -> To Workspace31/1
  oppose21/1 -> To Workspace34/1
  oppose20/1 -> To Workspace33/1
  oppose19/1 -> To Workspace32/1
  oppose17/1 -> To Workspace30/1
  oppose16/1 -> To Workspace29/1
  oppose14/1 -> To Workspace37/1
  oppose15/1 -> To Workspace38/1
  oppose13/1 -> To Workspace36/1
  oppose22/1 -> To Workspace35/1

== system CNcs5/CN/LMLN  03/03/01/oscillating PMC ==
  note: desired
      | eye accel
  note: original parameters:
      | tau3=30ms
      | tau2 = 35ms
      | fb gain = 1.1
  note: Robinson: PMC+ block
  note: motor
      | error
  note: efference
      | copy
  note: "Acceleration saturation" can be seen as a lookup table that
      | provides an acceleration for a given input velocity.  We then
      | use an integrator to convert the acceleration back to a velocity.
  note: From: Robinson DA, Gordon JL and Gordon SE
      | A model of smooth pursuit eye movements
      | Biological Cybernetics 55: 43-57,  1986
  note: By increasing feedback gain,
      | above 1.1 (about 2.2)
      | we can make this block oscillate at
      | a lower tau3 than it would otherwise.
  note: CN = 3.025
      | Norm = 1.1
  note: (Default=30ms, CN=40ms)
  note: (Default=35ms)
  note: (on = 0.0001)
      | (off = 0.0)
  desired eye vel : Inport  Port=1  LatchInput=off
  Sum : Sum  Inputs=-++  SaturateOnIntegerOverflow=on  InputSameDT=on
  Transfer Fcn2 : TransferFcn  Numerator=[pmcgain]  Denominator=[1 0]
  accel saturation : MATLABFcn  MATLABFcn=accsat
      mask Display: plot([-80 -4 4 80],[-120 -40 40 120], [0 0],[-120 120],[-80 80],[0 0])
  double pulse4 : FromWorkspace  VariableName=[0, t1, t1+.001, t1+d1, t1+d1+.001, t1+d1+.001+ipd, t1+d1+.001+ipd, t1+d1+.001+ipd+d2, t1+d1+.001+ipd+d2, 10000; 0, 0, p1, p1, 0, 0, p2, p2, 0, 0 ]'  mask{@1=825, @2=0, @3=.002, @4=.050, @5=-925, @6=.002}
      mask prompts: @1 "Pulse 1 Magnitude"; @2 "Time of Pulse 1 Onset"; @3 "Pulse 1 Duration"; @4 "Interpulse Delay"; @5 "Pulse 2 Magnitude"; @6 "Pulse 2 Duration"
      mask help: Double Pulse
      mask init:
      | p1=@1; t1=@2; d1=@3; ipd=@4; p2=@5; d2=@6;
      mask Display: disp('Double\nPulse')
  tau2 : TransportDelay  DelayTime=pmctau2/1000
  tau3 : TransportDelay  Orientation=left  DelayTime=pmctau3/1000
  velocity noise : simulink/Sources/Band-Limited White Noise  Orientation=up  Cov=[0.1]  Ts=0.1  seed=[23341]
  efference copy eye vel : Outport  InitialOutput=0
  wires:
  accel saturation/1 -> tau2/1
  tau2/1 -> Transfer Fcn2/1
  Sum/1 -> accel saturation/1
  tau3/1 -> Sum/1
  desired eye vel/1 -> Sum/2
  Transfer Fcn2/1 -> efference copy eye vel/1, tau3/1
  double pulse4/1 -> Sum/3

== system CNcs5/CN/LMLN  03/03/01/setmdlp ==

== system CNcs5/CN/LMLN  03/03/01/Fixation/30  ==
  note: init = 0
  note: init = 0
  note: 02/16/01
  note: The start of the input pulse causes the value on input 1 to be held starting when the leading
      | edge occurs, and this value remains latched until 'delay' seconds after the pulse ends (trailing edge).
  note: The two integration step delays before the S&H block's S/H (bottom) input insures
      | that the input value to be latched is available to theS&H block's top input
      | before the S&H block tries to 'hold'.
  note: Stretch the duration of an input pulse, latching it at its value at pulse onset.
  note: init Q = 0
  note: Changed from 1 to 2 delays
      | on 2/16/01 to provide insurance that
      | the signal at the S input will be available
  value(in) : Inport  Port=1  LatchInput=off
  " x/1000" : Constant  Orientation=up  Value=0.001
  Latch1 : simulink_extras/Flip Flops/S-R Flip-Flop  initial_condition=0
  Product : Product  SaturateOnIntegerOverflow=on  RndMeth=Zero  InputSameDT=on
  SampHold?2 : Subsystem
      mask Display: disp('S=L\nH=H')
  Variable Transport Delay : VariableTransportDelay  MaximumDelay=10
  leading edge detect : Subsystem
      mask Display: disp('Leading\nEdge Det')
  loop breaker2 : Memory
  loop breaker3 : Memory
  stretch : Constant  Value=prolong
  trailing edge detect : Subsystem
      mask Display: disp('Trailing\nEdge Det')
  value(out) : Outport  InitialOutput=0
  wires:
  " x/1000"/1 -> Product/2
  Product/1 -> Variable Transport Delay/2
  stretch/1 -> Product/1
  SampHold?2/1(output) -> value(out)/1
  trailing edge detect/1(out_1) -> Variable Transport Delay/1
  value(in)/1 -> SampHold?2/1(Input), trailing edge detect/1(in_1), leading edge detect/1(in_1)
  Latch1/1 -> loop breaker2/1
  loop breaker2/1 -> loop breaker3/1
  loop breaker3/1 -> SampHold?2/2(S/H?)
  leading edge detect/1(out_1) -> Latch1/1
  Variable Transport Delay/1 -> Latch1/2

== system CNcs5/CN/LMLN  03/03/01/Fixation/Boolify2 ==
  In1 : Inport  Port=1  LatchInput=off
  Abs2 : Abs  SaturateOnIntegerOverflow=on
  direction1 : Signum
  Out1 : Outport  InitialOutput=0
  wires:
  Abs2/1 -> direction1/1
  In1/1 -> Abs2/1
  direction1/1 -> Out1/1

== system CNcs5/CN/LMLN  03/03/01/IM CN-LMLN/Alexander's law ==
  note: Alexander's law
  ECPY [epospr] : Inport  Port=1  LatchInput=off
  TI : Inport  Port=2  LatchInput=off
  Boolify : Subsystem
      mask Display: disp('Boolify')
  Product : Product  SaturateOnIntegerOverflow=on  RndMeth=Zero  InputSameDT=on
  Product1 : Product  SaturateOnIntegerOverflow=on  RndMeth=Zero  InputSameDT=on
  Relational Operator : RelationalOperator  InputSameDT=on
  Relational Operator1 : RelationalOperator  Operator=<=  InputSameDT=on
  Sum : Sum  SaturateOnIntegerOverflow=on  InputSameDT=on
  Switch5 : Switch  SaturateOnIntegerOverflow=on  InputSameDT=on
  Switch6 : Switch  Threshold=.25  SaturateOnIntegerOverflow=on  InputSameDT=on
  Transfer Fcn : TransferFcn  Numerator=[5]  Denominator=[1 5]
  direction : Signum
  oppose1 : Constant  Orientation=up  Value=0
  oppose2 : Constant  Orientation=up  Value=0
  slope : Gain  Gain=slope  SaturateOnIntegerOverflow=on
  TIAL [tial] : Outport  InitialOutput=0
  wires:
  ECPY [epospr]/1 -> slope/1
  slope/1 -> Transfer Fcn/1
  Transfer Fcn/1 -> Sum/1
  Sum/1 -> Product1/1, Relational Operator/1, Product/2, Relational Operator1/1
  Relational Operator/1 -> Product1/2
  Product1/1 -> Switch5/1
  Relational Operator1/1 -> Product/1
  Product/1 -> Switch5/3
  oppose1/1 -> Relational Operator1/2, Relational Operator/2
  TI/1 -> direction/1, Sum/2, Boolify/1(TI)
  Switch5/1 -> Switch6/1
  Switch6/1 -> TIAL [tial]/1
  oppose2/1 -> Switch6/3
  direction/1 -> Switch5/2
  Boolify/1(Switch Control) -> Switch6/2

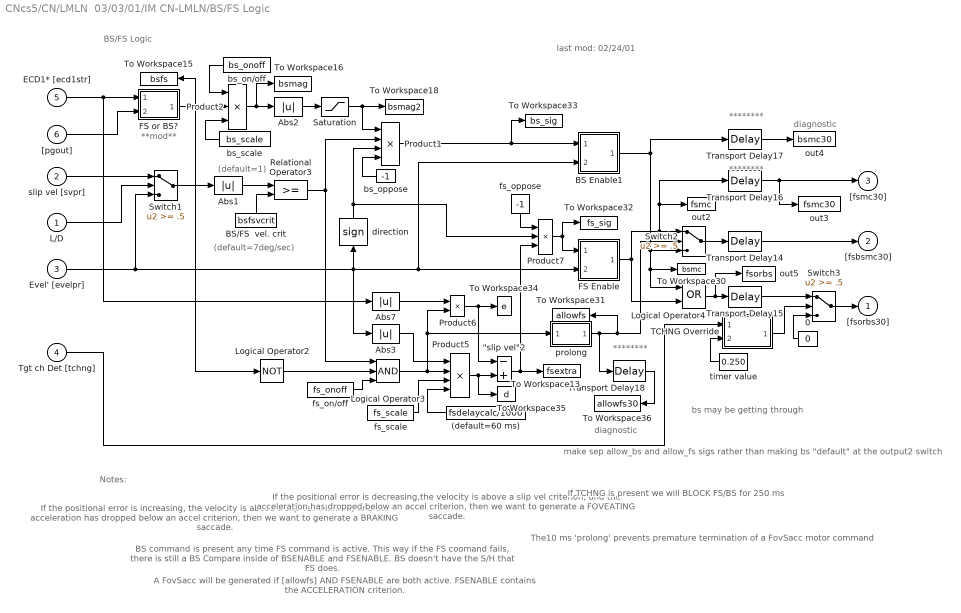
== system CNcs5/CN/LMLN  03/03/01/IM CN-LMLN/BS/FS Logic ==
  note: BS/FS Logic
  note: If the positional error is increasing, the velocity
      |  is above a slip vel criterion, and the acceleration
      | has dropped below an accel criterion, then we
      | want to generate a BRAKING saccade.
  note: If the positional error is decreasing,the velocity
      | is above a slip vel criterion, and the acceleration
      | has dropped below an accel criterion, then we
      | want to generate a FOVEATING saccade.
  note: last mod:
      | 02/24/01
  note: (default=7deg/sec)
  note: (default=1)
  note: If TCHNG is present we will BLOCK
      | FS/BS for 250 ms
  note: BS command is present any time FS command is active.  This way if the FS coomand fails, there is still a BS
      | Compare inside of BSENABLE and FSENABLE.  BS doesn't have the S/H that FS does.
  note: A FovSacc will be generated if [allowfs] AND FSENABLE are both active. FSENABLE contains the ACCELERATION criterion.
  note: Notes:
  note: The10 ms 'prolong' prevents premature
      | termination of a FovSacc motor command
  note: ********
  note: ********
  note: make sep allow_bs and allow_fs
      | sigs rather than making bs "default"
      | at the output2 switch
  note: bs may be getting through
  note: diagnostic
  note: diagnostic
  note: **mod**
  note: ********
  L/D : Inport  Port=1  LatchInput=off
  slip vel [svpr] : Inport  Port=2  LatchInput=off
  Evel' [evelpr] : Inport  Port=3  LatchInput=off
  Tgt ch Det [tchng] : Inport  Port=4  LatchInput=off
  ECD1* [ecd1str] : Inport  Port=5  LatchInput=off
  "[pgout]" : Inport  Port=6  LatchInput=off
  "\"slip vel\"2" : Sum  Inputs=-+  SaturateOnIntegerOverflow=on  InputSameDT=on
  (default=60 ms) : Constant  Orientation=left  Value=fsdelaycalc/1000
  0 : Constant  Orientation=left  Value=0
  Abs{1..3,7} (4 alike) : Abs  SaturateOnIntegerOverflow=on
  BS Enable1 : Subsystem
      mask Display: disp('BS\nEnab')
  BS/FS  vel. crit : Constant  Orientation=up  Value=bsfsvcrit
  FS Enable : Subsystem
      mask Display: disp('FS\nEnab')
  FS or BS? : Subsystem
      mask Display: disp('BS=1\nFS=0')
  Logical Operator2 : Logic  Operator=NOT  Inputs=1
  Logical Operator3 : Logic  Inputs=3
  Logical Operator4 : Logic  Operator=OR
  Product1 : Product  Inputs=4  SaturateOnIntegerOverflow=on  RndMeth=Zero  InputSameDT=on
  Product2 : Product  Inputs=3  SaturateOnIntegerOverflow=on  RndMeth=Zero  InputSameDT=on
  Product5 : Product  Inputs=4  SaturateOnIntegerOverflow=on  RndMeth=Zero  InputSameDT=on
  Product6 : Product  SaturateOnIntegerOverflow=on  RndMeth=Zero  InputSameDT=on
  Product7 : Product  Inputs=3  SaturateOnIntegerOverflow=on  RndMeth=Zero  InputSameDT=on
  Relational Operator3 : RelationalOperator  InputSameDT=on
  Saturation : Saturate  UpperLimit=2  LowerLimit=0
  Switch1 : Switch  Threshold=.5  SaturateOnIntegerOverflow=on  InputSameDT=on
  Switch2 : Switch  Threshold=.5  SaturateOnIntegerOverflow=on  InputSameDT=on
  Switch3 : Switch  Threshold=.5  SaturateOnIntegerOverflow=on  InputSameDT=on
  TCHNG Override : Subsystem
      mask Display: disp('TCHNG\nOverride')
  To Workspace13 : ToWorkspace  VariableName=fsextra  SaveFormat=Array
      settings: MaxDataPoints=10000
  To Workspace15 : ToWorkspace  VariableName=bsfs  SaveFormat=Array
      settings: MaxDataPoints=10000
  To Workspace16 : ToWorkspace  VariableName=bsmag  SaveFormat=Array
      settings: MaxDataPoints=10000
  To Workspace18 : ToWorkspace  VariableName=bsmag2  SaveFormat=Array
      settings: MaxDataPoints=10000
  To Workspace30 : ToWorkspace  VariableName=bsmc  SaveFormat=Array
      settings: MaxDataPoints=10000
  To Workspace31 : ToWorkspace  VariableName=allowfs  SaveFormat=Array
      settings: MaxDataPoints=10000
  To Workspace32 : ToWorkspace  VariableName=fs_sig  SaveFormat=Array
      settings: MaxDataPoints=10000
  To Workspace33 : ToWorkspace  VariableName=bs_sig  SaveFormat=Array
      settings: MaxDataPoints=10000
  To Workspace34 : ToWorkspace  VariableName=e  SaveFormat=Array
      settings: MaxDataPoints=10000
  To Workspace35 : ToWorkspace  VariableName=d  SaveFormat=Array
      settings: MaxDataPoints=10000
  To Workspace36 : ToWorkspace  VariableName=allowfs30  SaveFormat=Array
      settings: MaxDataPoints=10000
  Transport Delay{14..18} (5 alike) : TransportDelay  DelayTime=0.03
      mask Display: disp('30ms')
  bs_on/off : Constant  Orientation=left  Value=bs_onoff
  bs_oppose : Constant  Orientation=left  Value=-1
  bs_scale : Constant  Orientation=left  Value=bs_scale
  direction : Signum  Orientation=up
  fs_on/off : Constant  Value=fs_onoff
  fs_oppose : Constant  Orientation=down  Value=-1
  fs_scale : Constant  Value=fs_scale
  out2 : ToWorkspace  VariableName=fsmc  SaveFormat=Array
      settings: MaxDataPoints=100000
  out3 : ToWorkspace  VariableName=fsmc30  SaveFormat=Array
      settings: MaxDataPoints=100000
  out4 : ToWorkspace  VariableName=bsmc30  SaveFormat=Array
      settings: MaxDataPoints=100000
  out5 : ToWorkspace  VariableName=fsorbs  SaveFormat=Array
      settings: MaxDataPoints=100000
  prolong : Subsystem  mask{prolong=1}
      mask prompts: prolong "Prolong pulse by?  (msec)"
      mask Display: disp('prolong')
  timer value : Constant  Orientation=left  Value=0.250
  "[fsorbs30]" : Outport  InitialOutput=0
  "[fsbsmc30]" : Outport  Port=2  InitialOutput=0
  "[fsmc30]" : Outport  Port=3  InitialOutput=0
  wires:
  Abs2/1 -> Saturation/1
  FS or BS?/1(BS=1 FS=0) -> Product2/2, To Workspace15/1, Logical Operator2/1
  bs_on/off/1 -> Product2/1
  bs_scale/1 -> Product2/3
  Product2/1 -> Abs2/1, To Workspace16/1
  Saturation/1 -> Product1/1, To Workspace18/1
  L/D/1 -> Switch1/2
  slip vel [svpr]/1 -> Switch1/1
  Switch1/1 -> Abs1/1
  Evel' [evelpr]/1 -> Switch1/3, direction/1, BS Enable1/2("[evelpr]"), FS Enable/2("[evelpr]"), Abs3/1
  Relational Operator3/1 -> Logical Operator3/1, Product1/2
  "[pgout]"/1 -> FS or BS?/2(pgout)
  ECD1* [ecd1str]/1 -> FS or BS?/1(pos error [ecd1str]), Abs7/1
  BS/FS  vel. crit/1 -> Relational Operator3/2
  Abs1/1 -> Relational Operator3/1
  bs_oppose/1 -> Product1/4
  direction/1 -> Product1/3, Product7/2
  Logical Operator2/1 -> Logical Operator3/2
  (default=60 ms)/1 -> Product5/4
  Abs3/1 -> Product5/1
  Logical Operator3/1 -> Product5/2, Product6/2, prolong/1(value(in))
  fs_oppose/1 -> Product7/1
  Product5/1 -> "\"slip vel\"2"/2, To Workspace35/1
  "\"slip vel\"2"/1 -> Product7/3, To Workspace13/1
  Product7/1 -> FS Enable/1(fsprod), To Workspace32/1
  Abs7/1 -> Product6/1
  Product6/1 -> "\"slip vel\"2"/1, To Workspace34/1
  FS Enable/1("[fsmc]") -> Switch2/1, out2/1, Transport Delay16/1, Logical Operator4/2
  Switch2/1 -> Transport Delay14/1
  fs_scale/1 -> Product5/3
  fs_on/off/1 -> Logical Operator3/3
  Tgt ch Det [tchng]/1 -> TCHNG Override/1("[tchng]")
  timer value/1 -> TCHNG Override/2(timer dur)
  Transport Delay14/1 -> "[fsbsmc30]"/1
  Switch3/1 -> "[fsorbs30]"/1
  Transport Delay15/1 -> Switch3/1
  0/1 -> Switch3/3
  TCHNG Override/1(tchng sw) -> Switch3/2
  Transport Delay16/1 -> "[fsmc30]"/1, out3/1
  Product1/1 -> BS Enable1/1(bsprod), To Workspace33/1
  Transport Delay17/1 -> out4/1
  BS Enable1/1("[bsmc]") -> Switch2/3, Logical Operator4/1, To Workspace30/1, Transport Delay17/1
  Logical Operator4/1 -> Transport Delay15/1, out5/1
  prolong/1(value(out)) -> Switch2/2, To Workspace31/1, Transport Delay18/1
  Transport Delay18/1 -> To Workspace36/1

== system CNcs5/CN/LMLN  03/03/01/IM CN-LMLN/MdlPlnt+ ==
  note: Plant Model+
  note: last mod:
      | 01/31/00
  "[epossp]" : Inport  Port=1  LatchInput=off
  "[pgout]" : Inport  Port=2  LatchInput=off
  "\"Plant\"" : ZeroPole  Zeros=[ ]  Poles=[ -1/.18 -1/.007]  Gain=[1/.18 * 1/.007]
      mask Display: disp('2-pole\n"Plant"')
  Derivative : Derivative
      mask Display: disp('s')
  OMN2 : Subsystem
      mask Display: disp('<--tonic\nOMN2\n<--phasic')
  Transport Delay11 : TransportDelay  DelayTime=0.030
      mask Display: disp('30ms')
  Transport Delay12 : TransportDelay  DelayTime=0.050
      mask Display: disp('50ms')
  Transport Delay13 : TransportDelay  DelayTime=0.050
      mask Display: disp('50ms')
  "[ecpy80]" : Outport  InitialOutput=0
  "[imvel]" : Outport  Port=2  InitialOutput=0
  wires:
  Transport Delay13/1 -> "[imvel]"/1
  "[pgout]"/1 -> OMN2/2("[pgout]")
  "[epossp]"/1 -> OMN2/1("[epossp]")
  Derivative/1 -> Transport Delay13/1
  "\"Plant\""/1 -> Transport Delay12/1, Derivative/1
  Transport Delay11/1 -> "\"Plant\""/1
  OMN2/1(out_1) -> Transport Delay11/1
  Transport Delay12/1 -> "[ecpy80]"/1
